simulink model "Sollwertgenerator"  (R2015b)
settings: Solver=VariableStepAuto  StartTime=0.0  StopTime=10.0  RelTol=1e-3
values from neighbouring files (symbols this model uses):
  p = poly(-1*eye(4))    [Sollwert_Zusatz.m]    (also in Sollwertfilter.m = poly(lambda*eye(3)))
undefined symbols (not defined in the file or in its folder): parSollwertfilter
settings Model: Creator=J  LastModifiedBy=J

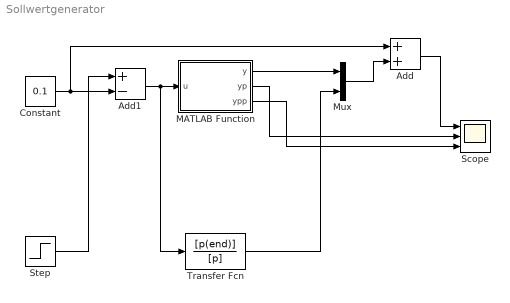
== system Sollwertgenerator ==
  Add : Sum
  Add1 : Sum  Inputs=+-
  Constant : Constant  Value=0.1
  MATLAB Function : MATLAB Function  TreatAsAtomicUnit=on  SystemSampleTime=parSollwertfilter.Ta
  Mux : Mux  Inputs=2
  Scope : Scope  NumInputPorts=3
  Step : Step  Before=0.1  After=0.2  SampleTime=0
  Transfer Fcn : TransferFcn  Numerator=[p(end)]  Denominator=[p]
  wires:
  Step/1 -> Add1/1
  Constant/1 -> Add/1, Add1/2
  Add1/1 -> Transfer Fcn/1, MATLAB Function/1(u)
  MATLAB Function/1(y) -> Mux/1
  MATLAB Function/2(yp) -> Scope/2
  MATLAB Function/3(ypp) -> Scope/3
  Mux/1 -> Add/2
  Add/1 -> Scope/1
  Transfer Fcn/1 -> Mux/2

== matlab function Sollwertgenerator/MATLAB Function ==
  settings: updateMethod=DISCRETE  sampleTime=parSollwertfilter.Ta
  data: u input; y output; yp output; ypp output; parSollwertfilter parameter
function [y,yp,ypp] = fcn(u, parSollwertfilter)
%#codegen
persistent x;

a=parSollwertfilter.a;
b=parSollwertfilter.b;
c=parSollwertfilter.c;
d=parSollwertfilter.d;

if(isempty(x))
    x0_Filter=parSollwertfilter.x0_Filter;
    x=x0_Filter;
end

yt= c*x + d*u;
y=yt(1);
yp=yt(2);
ypp=yt(3);

 x=a*x+b*u;
